simulink model "case7"  (R2024b)
settings: Solver=FixedStepAuto  StartTime=0  StopTime=1  FixedStep=1e-7  RelTol=1e-3
values from neighbouring files (symbols this model uses):
  SG_D_1_D = 0.01056    [IEEE9_case_parameters.m]    (also in case1_parameters.m; case2_parameters.m; case3_parameters.m; case4_parameters.m)
  SG_D_1_EnableSaturation = 0    [IEEE9_case_parameters.m]    (also in case1_parameters.m; case2_parameters.m; case3_parameters.m; case4_parameters.m)
  SG_D_1_f0 = 60    [IEEE9_case_parameters.m]    (also in case1_parameters.m; case2_parameters.m; case3_parameters.m; case4_parameters.m)
  SG_D_1_H = 7.5    [IEEE9_case_parameters.m]    (also in case1_parameters.m; case2_parameters.m; case3_parameters.m; case4_parameters.m)
  SG_D_1_K_A = 20    [IEEE9_case_parameters.m]    (also in case1_parameters.m; case2_parameters.m; case3_parameters.m; case4_parameters.m)
  SG_D_1_K_E = 1.000000e+1    (= 10)    [IEEE9_case_parameters.m]    (also in case1_parameters.m; case2_parameters.m; case3_parameters.m; case4_parameters.m)
  SG_D_1_K_F = 2.363    [IEEE9_case_parameters.m]    (also in case1_parameters.m; case2_parameters.m; case3_parameters.m; case4_parameters.m)
  SG_D_1_K_s = 0.5    [IEEE9_case_parameters.m]    (also in case1_parameters.m = 5; case2_parameters.m = 5; case3_parameters.m = 5; case4_parameters.m = 5)
  SG_D_1_R_a = 0.001088    [IEEE9_case_parameters.m]    (also in case1_parameters.m; case2_parameters.m; case3_parameters.m; case4_parameters.m)
  SG_D_1_S_A = 1    [IEEE9_case_parameters.m]    (also in case1_parameters.m; case2_parameters.m; case3_parameters.m; case4_parameters.m)
  SG_D_1_S_B = 0.103    [IEEE9_case_parameters.m]    (also in case1_parameters.m; case2_parameters.m; case3_parameters.m; case4_parameters.m)
  SG_D_1_S_N = 10.659857    [IEEE9_case_parameters.m]    (also in case1_parameters.m; case2_parameters.m; case3_parameters.m; case4_parameters.m)
  SG_D_1_SpeedPara = 200    [IEEE9_case_parameters.m]    (also in case1_parameters.m; case2_parameters.m; case3_parameters.m; case4_parameters.m)
  SG_D_1_T_0 = 0.720173    [IEEE9_case_parameters.m]    (also in case1_parameters.m = 0.755522; case2_parameters.m = 0.808931; case3_parameters.m = 0.869402; case4_parameters.m = 0.729316)
  SG_D_1_T_1 = 0.3    [IEEE9_case_parameters.m]    (also in case1_parameters.m; case2_parameters.m; case3_parameters.m; case4_parameters.m)
  SG_D_1_T_2 = 0.05    [IEEE9_case_parameters.m]    (also in case1_parameters.m; case2_parameters.m; case3_parameters.m; case4_parameters.m)
  SG_D_1_T_3 = 0.02    [IEEE9_case_parameters.m]    (also in case1_parameters.m; case2_parameters.m; case3_parameters.m; case4_parameters.m)
  SG_D_1_T_4 = 0.005    [IEEE9_case_parameters.m]    (also in case1_parameters.m; case2_parameters.m; case3_parameters.m; case4_parameters.m)
  SG_D_1_T_A = 0.02    [IEEE9_case_parameters.m]    (also in case1_parameters.m; case2_parameters.m; case3_parameters.m; case4_parameters.m)
  SG_D_1_T_dd = 8.000000e+0    (= 8)    [IEEE9_case_parameters.m]    (also in case1_parameters.m; case2_parameters.m; case3_parameters.m; case4_parameters.m)
  SG_D_1_T_ddd = 0.04    [IEEE9_case_parameters.m]    (also in case1_parameters.m; case2_parameters.m; case3_parameters.m; case4_parameters.m)
  SG_D_1_T_E = 0.314    [IEEE9_case_parameters.m]    (also in case1_parameters.m; case2_parameters.m; case3_parameters.m; case4_parameters.m)
  SG_D_1_T_F = 0.35    [IEEE9_case_parameters.m]    (also in case1_parameters.m; case2_parameters.m; case3_parameters.m; case4_parameters.m)
  SG_D_1_T_qd = 0.8    [IEEE9_case_parameters.m]    (also in case1_parameters.m; case2_parameters.m; case3_parameters.m; case4_parameters.m)
  SG_D_1_T_qdd = 0.02    [IEEE9_case_parameters.m]    (also in case1_parameters.m; case2_parameters.m; case3_parameters.m; case4_parameters.m)
  SG_D_1_T_speed = 0.1    [IEEE9_case_parameters.m]    (also in case1_parameters.m = 200; case2_parameters.m = 200; case3_parameters.m = 200; case4_parameters.m = 200)
  SG_D_1_T_w = 0.5    [IEEE9_case_parameters.m]    (also in case1_parameters.m; case2_parameters.m; case3_parameters.m; case4_parameters.m)
  SG_D_1_V_ref = 1.990276    [IEEE9_case_parameters.m]    (also in case1_parameters.m = 2.042296; case2_parameters.m = 2.051388; case3_parameters.m = 2.089584; case4_parameters.m = 2.01845)
  SG_D_1_w_ref = 376.991118    [IEEE9_case_parameters.m]    (also in case1_parameters.m; case2_parameters.m; case3_parameters.m; case4_parameters.m)
  SG_D_1_wb = 6.000000e+1    (= 60)    [IEEE9_case_parameters.m]    (also in case1_parameters.m; case2_parameters.m; case3_parameters.m; case4_parameters.m)
  SG_D_1_x_d = 1.9    [IEEE9_case_parameters.m]    (also in case1_parameters.m; case2_parameters.m; case3_parameters.m; case4_parameters.m)
  SG_D_1_x_dd = 0.302    [IEEE9_case_parameters.m]    (also in case1_parameters.m; case2_parameters.m; case3_parameters.m; case4_parameters.m)
  SG_D_1_x_ddd = 0.204    [IEEE9_case_parameters.m]    (also in case1_parameters.m; case2_parameters.m; case3_parameters.m; case4_parameters.m)
  SG_D_1_x_l = 0.05    [IEEE9_case_parameters.m]    (also in case1_parameters.m; case2_parameters.m; case3_parameters.m; case4_parameters.m)
  SG_D_1_x_q = 1.3    [IEEE9_case_parameters.m]    (also in case1_parameters.m; case2_parameters.m; case3_parameters.m; case4_parameters.m)
  SG_D_1_x_qd = 0.5    [IEEE9_case_parameters.m]    (also in case1_parameters.m; case2_parameters.m; case3_parameters.m; case4_parameters.m)
  SG_D_1_x_qdd = 0.3    [IEEE9_case_parameters.m]    (also in case1_parameters.m; case2_parameters.m; case3_parameters.m; case4_parameters.m)
  SG_D_2_D = 0.02    [IEEE9_case_parameters.m]    (also in case1_parameters.m; case2_parameters.m; case3_parameters.m; case4_parameters.m)
  SG_D_2_EnableSaturation = 0    [IEEE9_case_parameters.m]    (also in case1_parameters.m; case2_parameters.m; case3_parameters.m; case4_parameters.m)
  SG_D_2_f0 = 60    [IEEE9_case_parameters.m]    (also in case1_parameters.m; case2_parameters.m; case3_parameters.m; case4_parameters.m)
  SG_D_2_H = 8.000000e+0    (= 8)    [IEEE9_case_parameters.m]    (also in case1_parameters.m; case2_parameters.m; case3_parameters.m; case4_parameters.m)
  SG_D_2_K_A = 20    [IEEE9_case_parameters.m]    (also in case1_parameters.m; case2_parameters.m; case3_parameters.m; case4_parameters.m)
  SG_D_2_K_E = 1.000000e+1    (= 10)    [IEEE9_case_parameters.m]    (also in case1_parameters.m; case2_parameters.m; case3_parameters.m; case4_parameters.m)
  SG_D_2_K_F = 2.363    [IEEE9_case_parameters.m]    (also in case1_parameters.m; case2_parameters.m; case3_parameters.m; case4_parameters.m)
  SG_D_2_K_s = 0.5    [IEEE9_case_parameters.m]    (also in case1_parameters.m = 4; case2_parameters.m = 4; case3_parameters.m = 4; case4_parameters.m = 4)
  SG_D_2_R_a = 0.001088    [IEEE9_case_parameters.m]    (also in case1_parameters.m; case2_parameters.m; case3_parameters.m; case4_parameters.m)
  SG_D_2_S_A = 1    [IEEE9_case_parameters.m]    (also in case1_parameters.m; case2_parameters.m; case3_parameters.m; case4_parameters.m)
  SG_D_2_S_B = 0.103    [IEEE9_case_parameters.m]    (also in case1_parameters.m; case2_parameters.m; case3_parameters.m; case4_parameters.m)
  SG_D_2_S_N = 10.659857    [IEEE9_case_parameters.m]    (also in case1_parameters.m; case2_parameters.m; case3_parameters.m; case4_parameters.m)
  SG_D_2_SpeedPara = 200    [IEEE9_case_parameters.m]    (also in case1_parameters.m; case2_parameters.m; case3_parameters.m; case4_parameters.m)
  SG_D_2_T_0 = 1.632913    [IEEE9_case_parameters.m]    (also in case1_parameters.m = 1.632925; case2_parameters.m = 1.632915; case3_parameters.m = 1.632914; case4_parameters.m = 1.632927)
  SG_D_2_T_1 = 0.2    [IEEE9_case_parameters.m]    (also in case1_parameters.m; case2_parameters.m; case3_parameters.m; case4_parameters.m)
  SG_D_2_T_2 = 0.05    [IEEE9_case_parameters.m]    (also in case1_parameters.m; case2_parameters.m; case3_parameters.m; case4_parameters.m)
  SG_D_2_T_3 = 0.02    [IEEE9_case_parameters.m]    (also in case1_parameters.m; case2_parameters.m; case3_parameters.m; case4_parameters.m)
  SG_D_2_T_4 = 0.005    [IEEE9_case_parameters.m]    (also in case1_parameters.m; case2_parameters.m; case3_parameters.m; case4_parameters.m)
  SG_D_2_T_A = 0.02    [IEEE9_case_parameters.m]    (also in case1_parameters.m; case2_parameters.m; case3_parameters.m; case4_parameters.m)
  SG_D_2_T_dd = 7.9    [IEEE9_case_parameters.m]    (also in case1_parameters.m; case2_parameters.m; case3_parameters.m; case4_parameters.m)
  SG_D_2_T_ddd = 0.04    [IEEE9_case_parameters.m]    (also in case1_parameters.m; case2_parameters.m; case3_parameters.m; case4_parameters.m)
  SG_D_2_T_E = 0.314    [IEEE9_case_parameters.m]    (also in case1_parameters.m; case2_parameters.m; case3_parameters.m; case4_parameters.m)
  SG_D_2_T_F = 0.35    [IEEE9_case_parameters.m]    (also in case1_parameters.m; case2_parameters.m; case3_parameters.m; case4_parameters.m)
  SG_D_2_T_qd = 0.8    [IEEE9_case_parameters.m]    (also in case1_parameters.m; case2_parameters.m; case3_parameters.m; case4_parameters.m)
  SG_D_2_T_qdd = 0.015    [IEEE9_case_parameters.m]    (also in case1_parameters.m; case2_parameters.m; case3_parameters.m; case4_parameters.m)
  SG_D_2_T_speed = 0.1    [IEEE9_case_parameters.m]    (also in case1_parameters.m = 150; case2_parameters.m = 150; case3_parameters.m = 150; case4_parameters.m = 150)
  SG_D_2_T_w = 0.35    [IEEE9_case_parameters.m]    (also in case1_parameters.m; case2_parameters.m; case3_parameters.m; case4_parameters.m)
  SG_D_2_V_ref = 2.58547    [IEEE9_case_parameters.m]    (also in case1_parameters.m = 2.597896; case2_parameters.m = 2.587136; case3_parameters.m = 2.586042; case4_parameters.m = 2.599679)
  SG_D_2_w_ref = 376.991118    [IEEE9_case_parameters.m]    (also in case1_parameters.m; case2_parameters.m; case3_parameters.m; case4_parameters.m)
  SG_D_2_wb = 6.000000e+1    (= 60)    [IEEE9_case_parameters.m]    (also in case1_parameters.m; case2_parameters.m; case3_parameters.m; case4_parameters.m)
  SG_D_2_x_d = 1.8    [IEEE9_case_parameters.m]    (also in case1_parameters.m; case2_parameters.m; case3_parameters.m; case4_parameters.m)
  SG_D_2_x_dd = 0.302    [IEEE9_case_parameters.m]    (also in case1_parameters.m; case2_parameters.m; case3_parameters.m; case4_parameters.m)
  SG_D_2_x_ddd = 0.204    [IEEE9_case_parameters.m]    (also in case1_parameters.m; case2_parameters.m; case3_parameters.m; case4_parameters.m)
  SG_D_2_x_l = 0.05    [IEEE9_case_parameters.m]    (also in case1_parameters.m; case2_parameters.m; case3_parameters.m; case4_parameters.m)
  SG_D_2_x_q = 1.25    [IEEE9_case_parameters.m]    (also in case1_parameters.m; case2_parameters.m; case3_parameters.m; case4_parameters.m)
  SG_D_2_x_qd = 0.5    [IEEE9_case_parameters.m]    (also in case1_parameters.m; case2_parameters.m; case3_parameters.m; case4_parameters.m)
  SG_D_2_x_qdd = 0.3    [IEEE9_case_parameters.m]    (also in case1_parameters.m; case2_parameters.m; case3_parameters.m; case4_parameters.m)
  SG_D_3_D = 0.02    [IEEE9_case_parameters.m]    (also in case1_parameters.m; case2_parameters.m; case3_parameters.m; case4_parameters.m)
  SG_D_3_EnableSaturation = 0    [IEEE9_case_parameters.m]    (also in case1_parameters.m; case2_parameters.m; case3_parameters.m; case4_parameters.m)
  SG_D_3_f0 = 60    [IEEE9_case_parameters.m]    (also in case1_parameters.m; case2_parameters.m; case3_parameters.m; case4_parameters.m)
  SG_D_3_H = 7.7    [IEEE9_case_parameters.m]    (also in case1_parameters.m; case2_parameters.m; case3_parameters.m; case4_parameters.m)
  SG_D_3_K_A = 20    [IEEE9_case_parameters.m]    (also in case1_parameters.m; case2_parameters.m; case3_parameters.m; case4_parameters.m)
  SG_D_3_K_E = 1.000000e+1    (= 10)    [IEEE9_case_parameters.m]    (also in case1_parameters.m; case2_parameters.m; case3_parameters.m; case4_parameters.m)
  SG_D_3_K_F = 2.363    [IEEE9_case_parameters.m]    (also in case1_parameters.m; case2_parameters.m; case3_parameters.m; case4_parameters.m)
  SG_D_3_K_s = 0.2    [IEEE9_case_parameters.m]    (also in case1_parameters.m = 2; case2_parameters.m = 2; case3_parameters.m = 2; case4_parameters.m = 2)
  SG_D_3_R_a = 0.001088    [IEEE9_case_parameters.m]    (also in case1_parameters.m; case2_parameters.m; case3_parameters.m; case4_parameters.m)
  SG_D_3_S_A = 1    [IEEE9_case_parameters.m]    (also in case1_parameters.m; case2_parameters.m; case3_parameters.m; case4_parameters.m)
  SG_D_3_S_B = 0.103    [IEEE9_case_parameters.m]    (also in case1_parameters.m; case2_parameters.m; case3_parameters.m; case4_parameters.m)
  SG_D_3_S_N = 10.659857    [IEEE9_case_parameters.m]    (also in case1_parameters.m; case2_parameters.m; case3_parameters.m; case4_parameters.m)
  SG_D_3_SpeedPara = 200    [IEEE9_case_parameters.m]    (also in case1_parameters.m; case2_parameters.m; case3_parameters.m; case4_parameters.m)
  SG_D_3_T_0 = 0.850788    [IEEE9_case_parameters.m]    (also in case1_parameters.m = 0.850786; case2_parameters.m = 0.850787; case3_parameters.m; case4_parameters.m = 0.850786)
  SG_D_3_T_1 = 0.2    [IEEE9_case_parameters.m]    (also in case1_parameters.m; case2_parameters.m; case3_parameters.m; case4_parameters.m)
  SG_D_3_T_2 = 0.05    [IEEE9_case_parameters.m]    (also in case1_parameters.m; case2_parameters.m; case3_parameters.m; case4_parameters.m)
  SG_D_3_T_3 = 0.02    [IEEE9_case_parameters.m]    (also in case1_parameters.m; case2_parameters.m; case3_parameters.m; case4_parameters.m)
  SG_D_3_T_4 = 0.005    [IEEE9_case_parameters.m]    (also in case1_parameters.m; case2_parameters.m; case3_parameters.m; case4_parameters.m)
  SG_D_3_T_A = 0.02    [IEEE9_case_parameters.m]    (also in case1_parameters.m; case2_parameters.m; case3_parameters.m; case4_parameters.m)
  SG_D_3_T_dd = 8.1    [IEEE9_case_parameters.m]    (also in case1_parameters.m; case2_parameters.m; case3_parameters.m; case4_parameters.m)
  SG_D_3_T_ddd = 0.04    [IEEE9_case_parameters.m]    (also in case1_parameters.m; case2_parameters.m; case3_parameters.m; case4_parameters.m)
  SG_D_3_T_E = 0.314    [IEEE9_case_parameters.m]    (also in case1_parameters.m; case2_parameters.m; case3_parameters.m; case4_parameters.m)
  SG_D_3_T_F = 0.35    [IEEE9_case_parameters.m]    (also in case1_parameters.m; case2_parameters.m; case3_parameters.m; case4_parameters.m)
  SG_D_3_T_qd = 0.8    [IEEE9_case_parameters.m]    (also in case1_parameters.m; case2_parameters.m; case3_parameters.m; case4_parameters.m)
  SG_D_3_T_qdd = 0.015    [IEEE9_case_parameters.m]    (also in case1_parameters.m; case2_parameters.m; case3_parameters.m; case4_parameters.m)
  SG_D_3_T_speed = 0.1    [IEEE9_case_parameters.m]    (also in case1_parameters.m = 180; case2_parameters.m = 180; case3_parameters.m = 180; case4_parameters.m = 180)
  SG_D_3_T_w = 0.4    [IEEE9_case_parameters.m]    (also in case1_parameters.m; case2_parameters.m; case3_parameters.m; case4_parameters.m)
  SG_D_3_V_ref = 1.892727    [IEEE9_case_parameters.m]    (also in case1_parameters.m = 1.906439; case2_parameters.m = 1.895535; case3_parameters.m = 1.892105; case4_parameters.m = 1.906598)
  SG_D_3_w_ref = 376.991118    [IEEE9_case_parameters.m]    (also in case1_parameters.m; case2_parameters.m; case3_parameters.m; case4_parameters.m)
  SG_D_3_wb = 6.000000e+1    (= 60)    [IEEE9_case_parameters.m]    (also in case1_parameters.m; case2_parameters.m; case3_parameters.m; case4_parameters.m)
  SG_D_3_x_d = 1.85    [IEEE9_case_parameters.m]    (also in case1_parameters.m; case2_parameters.m; case3_parameters.m; case4_parameters.m)
  SG_D_3_x_dd = 0.302    [IEEE9_case_parameters.m]    (also in case1_parameters.m; case2_parameters.m; case3_parameters.m; case4_parameters.m)
  SG_D_3_x_ddd = 0.204    [IEEE9_case_parameters.m]    (also in case1_parameters.m; case2_parameters.m; case3_parameters.m; case4_parameters.m)
  SG_D_3_x_l = 0.05    [IEEE9_case_parameters.m]    (also in case1_parameters.m; case2_parameters.m; case3_parameters.m; case4_parameters.m)
  SG_D_3_x_q = 1.2    [IEEE9_case_parameters.m]    (also in case1_parameters.m; case2_parameters.m; case3_parameters.m; case4_parameters.m)
  SG_D_3_x_qd = 0.5    [IEEE9_case_parameters.m]    (also in case1_parameters.m; case2_parameters.m; case3_parameters.m; case4_parameters.m)
  SG_D_3_x_qdd = 0.3    [IEEE9_case_parameters.m]    (also in case1_parameters.m; case2_parameters.m; case3_parameters.m; case4_parameters.m)
(part 4 of 12)

== system case7/AC_1/d_vq_bus_7_block ==
  note: d_vq_bus_7 in case7
      | $2106.09563369148\,\mathrm{iq}_{\mathrm{bus},7}-376.991118430775\,\mathrm{vd}_{\mathrm{bus},7}$
      | Automatically generated on 2025-10-31 19:27:14 .
  Alge_iq_bus_7_6c77e : Inport
  State_vd_bus_7_c0edf : Inport  Port=2
  Constant_2106.09563369148_c22c3 : Constant  Value=2106.09563369148
  Constant_376.991118430775_b78ad : Constant  Value=376.991118430775
  Product_08e92 : Product
  Product_2e90c : Product
  Subtract_efe12 : Sum  Inputs=+-
  Blockout_d_vq_bus_7_c9af2 : Outport
  wires:
  Constant_2106.09563369148_c22c3/1 -> Product_2e90c/1
  Product_08e92/1 -> Subtract_efe12/2
  Alge_iq_bus_7_6c77e/1 -> Product_2e90c/2
  Constant_376.991118430775_b78ad/1 -> Product_08e92/1
  Subtract_efe12/1 -> Blockout_d_vq_bus_7_c9af2/1
  State_vd_bus_7_c0edf/1 -> Product_08e92/2
  Product_2e90c/1 -> Subtract_efe12/1

== system case7/AC_1/d_vq_bus_8_block ==
  note: d_vq_bus_8 in case7
      | $1657.10381727813\,\mathrm{iq}_{\mathrm{bus},8}-376.991118430775\,\mathrm{vd}_{\mathrm{bus},8}$
      | Automatically generated on 2025-10-31 19:27:16 .
  Alge_iq_bus_8_b3710 : Inport
  State_vd_bus_8_12b43 : Inport  Port=2
  Constant_1657.10381727813_46e6f : Constant  Value=1657.10381727813
  Constant_376.991118430775_a10c9 : Constant  Value=376.991118430775
  Product_577b0 : Product
  Product_c9932 : Product
  Subtract_67862 : Sum  Inputs=+-
  Blockout_d_vq_bus_8_09663 : Outport
  wires:
  Constant_1657.10381727813_46e6f/1 -> Product_577b0/1
  Constant_376.991118430775_a10c9/1 -> Product_c9932/1
  Alge_iq_bus_8_b3710/1 -> Product_577b0/2
  State_vd_bus_8_12b43/1 -> Product_c9932/2
  Product_577b0/1 -> Subtract_67862/1
  Product_c9932/1 -> Subtract_67862/2
  Subtract_67862/1 -> Blockout_d_vq_bus_8_09663/1

== system case7/AC_1/d_vq_bus_9_block ==
  note: d_vq_bus_9 in case7
      | $1564.27849971276\,\mathrm{iq}_{\mathrm{bus},9}-376.991118430775\,\mathrm{vd}_{\mathrm{bus},9}$
      | Automatically generated on 2025-10-31 19:27:19 .
  Alge_iq_bus_9_a8f96 : Inport
  State_vd_bus_9_2f8b2 : Inport  Port=2
  Constant_1564.27849971276_a9894 : Constant  Value=1564.27849971276
  Constant_376.991118430775_a939a : Constant  Value=376.991118430775
  Product_678dc : Product
  Product_f03d7 : Product
  Subtract_bc8b5 : Sum  Inputs=+-
  Blockout_d_vq_bus_9_31261 : Outport
  wires:
  Constant_1564.27849971276_a9894/1 -> Product_f03d7/1
  Constant_376.991118430775_a939a/1 -> Product_678dc/1
  Alge_iq_bus_9_a8f96/1 -> Product_f03d7/2
  State_vd_bus_9_2f8b2/1 -> Product_678dc/2
  Product_f03d7/1 -> Subtract_bc8b5/1
  Product_678dc/1 -> Subtract_bc8b5/2
  Subtract_bc8b5/1 -> Blockout_d_vq_bus_9_31261/1

== system case7/AC_1/id_bus_1_block ==
  note: id_bus_1 in case7
      | $\mathrm{id}_{\mathrm{SG},D,1}-\mathrm{id}_{\mathrm{line},1,4}$
      | Automatically generated on 2025-10-31 19:28:04 .
  Input_id_SG_D_1_eabc6 : Inport
  State_id_line_1_4_aab97 : Inport  Port=2
  Subtract_4393a : Sum  Inputs=+-
  Blockout_id_bus_1_e0036 : Outport
  wires:
  Input_id_SG_D_1_eabc6/1 -> Subtract_4393a/1
  State_id_line_1_4_aab97/1 -> Subtract_4393a/2
  Subtract_4393a/1 -> Blockout_id_bus_1_e0036/1

== system case7/AC_1/id_bus_2_block ==
  note: id_bus_2 in case7
      | $\mathrm{id}_{\mathrm{SG},D,2}+\mathrm{id}_{\mathrm{line},8,2}$
      | Automatically generated on 2025-10-31 19:28:08 .
  Input_id_SG_D_2_cbeb2 : Inport
  State_id_line_8_2_ddc5d : Inport  Port=2
  Add_5b75e : Sum
  Blockout_id_bus_2_1dfd8 : Outport
  wires:
  Input_id_SG_D_2_cbeb2/1 -> Add_5b75e/1
  State_id_line_8_2_ddc5d/1 -> Add_5b75e/2
  Add_5b75e/1 -> Blockout_id_bus_2_1dfd8/1

== system case7/AC_1/id_bus_3_block ==
  note: id_bus_3 in case7
      | $\mathrm{id}_{\mathrm{SG},D,3}-\mathrm{id}_{\mathrm{line},3,6}$
      | Automatically generated on 2025-10-31 19:28:12 .
  Input_id_SG_D_3_5761d : Inport
  State_id_line_3_6_23ff0 : Inport  Port=2
  Subtract_5b783 : Sum  Inputs=+-
  Blockout_id_bus_3_ffcf5 : Outport
  wires:
  Input_id_SG_D_3_5761d/1 -> Subtract_5b783/1
  State_id_line_3_6_23ff0/1 -> Subtract_5b783/2
  Subtract_5b783/1 -> Blockout_id_bus_3_ffcf5/1

== system case7/AC_1/id_bus_4_block ==
  note: id_bus_4 in case7
      | $\mathrm{id}_{\mathrm{line},1,4}-\mathrm{id}_{\mathrm{line},4,5}+\mathrm{id}_{\mathrm{line},9,4}$
      | Automatically generated on 2025-10-31 19:28:14 .
  State_id_line_1_4_3a3fb : Inport
  State_id_line_4_5_64512 : Inport  Port=2
  State_id_line_9_4_0d956 : Inport  Port=3
  Add_d04b2 : Sum
  Subtract_5520f : Sum  Inputs=+-
  Blockout_id_bus_4_096f4 : Outport
  wires:
  State_id_line_9_4_0d956/1 -> Add_d04b2/2
  State_id_line_1_4_3a3fb/1 -> Subtract_5520f/1
  State_id_line_4_5_64512/1 -> Subtract_5520f/2
  Subtract_5520f/1 -> Add_d04b2/1
  Add_d04b2/1 -> Blockout_id_bus_4_096f4/1

== system case7/AC_1/id_bus_5_block ==
  note: id_bus_5 in case7
      | $\mathrm{id}_{\mathrm{line},4,5}-\mathrm{id}_{\mathrm{load},5}-\mathrm{id}_{\mathrm{line},5,6}$
      | Automatically generated on 2025-10-31 19:28:16 .
  State_id_load_5_a1fc8 : Inport
  State_id_line_4_5_aeb7d : Inport  Port=2
  State_id_line_5_6_7e5e7 : Inport  Port=3
  Add_d6f2a : Sum
  Constant_-1_2d1af : Constant  Value=-1
  Product_7594e : Product
  Subtract_9d0cf : Sum  Inputs=+-
  Blockout_id_bus_5_d8728 : Outport
  wires:
  Subtract_9d0cf/1 -> Blockout_id_bus_5_d8728/1
  State_id_line_4_5_aeb7d/1 -> Add_d6f2a/2
  Constant_-1_2d1af/1 -> Product_7594e/1
  Add_d6f2a/1 -> Subtract_9d0cf/1
  State_id_load_5_a1fc8/1 -> Product_7594e/2
  Product_7594e/1 -> Add_d6f2a/1
  State_id_line_5_6_7e5e7/1 -> Subtract_9d0cf/2

== system case7/AC_1/id_bus_6_block ==
  note: id_bus_6 in case7
      | $\mathrm{id}_{\mathrm{line},3,6}+\mathrm{id}_{\mathrm{line},5,6}-\mathrm{id}_{\mathrm{line},6,7}$
      | Automatically generated on 2025-10-31 19:28:18 .
  State_id_line_3_6_b6780 : Inport
  State_id_line_5_6_2d0d9 : Inport  Port=2
  State_id_line_6_7_41759 : Inport  Port=3
  Add_e2ec4 : Sum
  Subtract_1dfb6 : Sum  Inputs=+-
  Blockout_id_bus_6_34f1f : Outport
  wires:
  State_id_line_6_7_41759/1 -> Subtract_1dfb6/2
  State_id_line_3_6_b6780/1 -> Add_e2ec4/1
  State_id_line_5_6_2d0d9/1 -> Add_e2ec4/2
  Add_e2ec4/1 -> Subtract_1dfb6/1
  Subtract_1dfb6/1 -> Blockout_id_bus_6_34f1f/1

== system case7/AC_1/id_bus_7_block ==
  note: id_bus_7 in case7
      | $\mathrm{id}_{\mathrm{line},6,7}-\mathrm{id}_{\mathrm{load},7}-\mathrm{id}_{\mathrm{line},7,8}$
      | Automatically generated on 2025-10-31 19:28:20 .
  State_id_load_7_264fa : Inport
  State_id_line_6_7_22f92 : Inport  Port=2
  State_id_line_7_8_244b4 : Inport  Port=3
  Add_ca084 : Sum
  Constant_-1_8693b : Constant  Value=-1
  Product_5b7d9 : Product
  Subtract_8746d : Sum  Inputs=+-
  Blockout_id_bus_7_f40f2 : Outport
  wires:
  Subtract_8746d/1 -> Blockout_id_bus_7_f40f2/1
  State_id_line_6_7_22f92/1 -> Add_ca084/2
  Constant_-1_8693b/1 -> Product_5b7d9/1
  Add_ca084/1 -> Subtract_8746d/1
  State_id_load_7_264fa/1 -> Product_5b7d9/2
  Product_5b7d9/1 -> Add_ca084/1
  State_id_line_7_8_244b4/1 -> Subtract_8746d/2

== system case7/AC_1/id_bus_8_block ==
  note: id_bus_8 in case7
      | $\mathrm{id}_{\mathrm{line},7,8}-\mathrm{id}_{\mathrm{line},8,2}-\mathrm{id}_{\mathrm{line},8,9}$
      | Automatically generated on 2025-10-31 19:28:23 .
  State_id_line_7_8_e0e98 : Inport
  State_id_line_8_2_e2197 : Inport  Port=2
  State_id_line_8_9_6c8e7 : Inport  Port=3
  Subtract_1c8c3 : Sum  Inputs=+-
  Subtract_aa105 : Sum  Inputs=+-
  Blockout_id_bus_8_dcf1d : Outport
  wires:
  State_id_line_8_9_6c8e7/1 -> Subtract_aa105/2
  State_id_line_7_8_e0e98/1 -> Subtract_1c8c3/1
  State_id_line_8_2_e2197/1 -> Subtract_1c8c3/2
  Subtract_1c8c3/1 -> Subtract_aa105/1
  Subtract_aa105/1 -> Blockout_id_bus_8_dcf1d/1

== system case7/AC_1/id_bus_9_block ==
  note: id_bus_9 in case7
      | $\mathrm{id}_{\mathrm{line},8,9}-\mathrm{id}_{\mathrm{load},9}-\mathrm{id}_{\mathrm{line},9,4}$
      | Automatically generated on 2025-10-31 19:28:25 .
  State_id_load_9_bf11f : Inport
  State_id_line_8_9_50722 : Inport  Port=2
  State_id_line_9_4_40117 : Inport  Port=3
  Add_348e1 : Sum
  Constant_-1_413c0 : Constant  Value=-1
  Product_27b0f : Product
  Subtract_5cca6 : Sum  Inputs=+-
  Blockout_id_bus_9_4ad6a : Outport
  wires:
  Subtract_5cca6/1 -> Blockout_id_bus_9_4ad6a/1
  State_id_line_8_9_50722/1 -> Add_348e1/2
  Constant_-1_413c0/1 -> Product_27b0f/1
  Add_348e1/1 -> Subtract_5cca6/1
  State_id_load_9_bf11f/1 -> Product_27b0f/2
  Product_27b0f/1 -> Add_348e1/1
  State_id_line_9_4_40117/1 -> Subtract_5cca6/2

== system case7/AC_1/iq_bus_1_block ==
  note: iq_bus_1 in case7
      | $\mathrm{iq}_{\mathrm{SG},D,1}-\mathrm{iq}_{\mathrm{line},1,4}$
      | Automatically generated on 2025-10-31 19:28:05 .
  Input_iq_SG_D_1_419da : Inport
  State_iq_line_1_4_cde6a : Inport  Port=2
  Subtract_68868 : Sum  Inputs=+-
  Blockout_iq_bus_1_23a9f : Outport
  wires:
  Input_iq_SG_D_1_419da/1 -> Subtract_68868/1
  State_iq_line_1_4_cde6a/1 -> Subtract_68868/2
  Subtract_68868/1 -> Blockout_iq_bus_1_23a9f/1

== system case7/AC_1/iq_bus_2_block ==
  note: iq_bus_2 in case7
      | $\mathrm{iq}_{\mathrm{SG},D,2}+\mathrm{iq}_{\mathrm{line},8,2}$
      | Automatically generated on 2025-10-31 19:28:09 .
  Input_iq_SG_D_2_9dccc : Inport
  State_iq_line_8_2_f6d21 : Inport  Port=2
  Add_07ce0 : Sum
  Blockout_iq_bus_2_f07a2 : Outport
  wires:
  Input_iq_SG_D_2_9dccc/1 -> Add_07ce0/1
  State_iq_line_8_2_f6d21/1 -> Add_07ce0/2
  Add_07ce0/1 -> Blockout_iq_bus_2_f07a2/1

== system case7/AC_1/iq_bus_3_block ==
  note: iq_bus_3 in case7
      | $\mathrm{iq}_{\mathrm{SG},D,3}-\mathrm{iq}_{\mathrm{line},3,6}$
      | Automatically generated on 2025-10-31 19:28:13 .
  Input_iq_SG_D_3_c42e5 : Inport
  State_iq_line_3_6_82adc : Inport  Port=2
  Subtract_76832 : Sum  Inputs=+-
  Blockout_iq_bus_3_7920f : Outport
  wires:
  Input_iq_SG_D_3_c42e5/1 -> Subtract_76832/1
  State_iq_line_3_6_82adc/1 -> Subtract_76832/2
  Subtract_76832/1 -> Blockout_iq_bus_3_7920f/1

== system case7/AC_1/iq_bus_4_block ==
  note: iq_bus_4 in case7
      | $\mathrm{iq}_{\mathrm{line},1,4}-\mathrm{iq}_{\mathrm{line},4,5}+\mathrm{iq}_{\mathrm{line},9,4}$
      | Automatically generated on 2025-10-31 19:28:15 .
  State_iq_line_1_4_6e840 : Inport
  State_iq_line_4_5_67a6b : Inport  Port=2
  State_iq_line_9_4_bc136 : Inport  Port=3
  Add_d19bc : Sum
  Subtract_43078 : Sum  Inputs=+-
  Blockout_iq_bus_4_5b7f0 : Outport
  wires:
  State_iq_line_1_4_6e840/1 -> Subtract_43078/1
  State_iq_line_4_5_67a6b/1 -> Subtract_43078/2
  Subtract_43078/1 -> Add_d19bc/1
  State_iq_line_9_4_bc136/1 -> Add_d19bc/2
  Add_d19bc/1 -> Blockout_iq_bus_4_5b7f0/1

== system case7/AC_1/iq_bus_5_block ==
  note: iq_bus_5 in case7
      | $\mathrm{iq}_{\mathrm{line},4,5}-\mathrm{iq}_{\mathrm{load},5}-\mathrm{iq}_{\mathrm{line},5,6}$
      | Automatically generated on 2025-10-31 19:28:17 .
  State_iq_load_5_f86bc : Inport
  State_iq_line_4_5_93363 : Inport  Port=2
  State_iq_line_5_6_43169 : Inport  Port=3
  Add_32bb9 : Sum
  Constant_-1_d5412 : Constant  Value=-1
  Product_94716 : Product
  Subtract_7acf6 : Sum  Inputs=+-
  Blockout_iq_bus_5_1d005 : Outport
  wires:
  Subtract_7acf6/1 -> Blockout_iq_bus_5_1d005/1
  State_iq_line_4_5_93363/1 -> Add_32bb9/2
  Constant_-1_d5412/1 -> Product_94716/1
  State_iq_load_5_f86bc/1 -> Product_94716/2
  Product_94716/1 -> Add_32bb9/1
  Add_32bb9/1 -> Subtract_7acf6/1
  State_iq_line_5_6_43169/1 -> Subtract_7acf6/2

== system case7/AC_1/iq_bus_6_block ==
  note: iq_bus_6 in case7
      | $\mathrm{iq}_{\mathrm{line},3,6}+\mathrm{iq}_{\mathrm{line},5,6}-\mathrm{iq}_{\mathrm{line},6,7}$
      | Automatically generated on 2025-10-31 19:28:19 .
  State_iq_line_3_6_53eaa : Inport
  State_iq_line_5_6_87c1e : Inport  Port=2
  State_iq_line_6_7_e327a : Inport  Port=3
  Add_19bb9 : Sum
  Subtract_e9880 : Sum  Inputs=+-
  Blockout_iq_bus_6_0cb61 : Outport
  wires:
  State_iq_line_3_6_53eaa/1 -> Add_19bb9/1
  State_iq_line_5_6_87c1e/1 -> Add_19bb9/2
  Add_19bb9/1 -> Subtract_e9880/1
  State_iq_line_6_7_e327a/1 -> Subtract_e9880/2
  Subtract_e9880/1 -> Blockout_iq_bus_6_0cb61/1

== system case7/AC_1/iq_bus_7_block ==
  note: iq_bus_7 in case7
      | $\mathrm{iq}_{\mathrm{line},6,7}-\mathrm{iq}_{\mathrm{load},7}-\mathrm{iq}_{\mathrm{line},7,8}$
      | Automatically generated on 2025-10-31 19:28:22 .
  State_iq_load_7_cacac : Inport
  State_iq_line_6_7_1e244 : Inport  Port=2
  State_iq_line_7_8_8c678 : Inport  Port=3
  Add_08d5a : Sum
  Constant_-1_82b11 : Constant  Value=-1
  Product_c20ef : Product
  Subtract_827af : Sum  Inputs=+-
  Blockout_iq_bus_7_f78e5 : Outport
  wires:
  Subtract_827af/1 -> Blockout_iq_bus_7_f78e5/1
  State_iq_line_6_7_1e244/1 -> Add_08d5a/2
  Constant_-1_82b11/1 -> Product_c20ef/1
  State_iq_load_7_cacac/1 -> Product_c20ef/2
  Product_c20ef/1 -> Add_08d5a/1
  Add_08d5a/1 -> Subtract_827af/1
  State_iq_line_7_8_8c678/1 -> Subtract_827af/2

== system case7/AC_1/iq_bus_8_block ==
  note: iq_bus_8 in case7
      | $\mathrm{iq}_{\mathrm{line},7,8}-\mathrm{iq}_{\mathrm{line},8,2}-\mathrm{iq}_{\mathrm{line},8,9}$
      | Automatically generated on 2025-10-31 19:28:24 .
  State_iq_line_7_8_8361f : Inport
  State_iq_line_8_2_4ece4 : Inport  Port=2
  State_iq_line_8_9_62274 : Inport  Port=3
  Subtract_aaa9d : Sum  Inputs=+-
  Subtract_ba02c : Sum  Inputs=+-
  Blockout_iq_bus_8_3d53c : Outport
  wires:
  State_iq_line_7_8_8361f/1 -> Subtract_aaa9d/1
  State_iq_line_8_2_4ece4/1 -> Subtract_aaa9d/2
  Subtract_aaa9d/1 -> Subtract_ba02c/1
  State_iq_line_8_9_62274/1 -> Subtract_ba02c/2
  Subtract_ba02c/1 -> Blockout_iq_bus_8_3d53c/1

== system case7/AC_1/iq_bus_9_block ==
  note: iq_bus_9 in case7
      | $\mathrm{iq}_{\mathrm{line},8,9}-\mathrm{iq}_{\mathrm{load},9}-\mathrm{iq}_{\mathrm{line},9,4}$
      | Automatically generated on 2025-10-31 19:28:26 .
  State_iq_load_9_c0b16 : Inport
  State_iq_line_8_9_e9f4e : Inport  Port=2
  State_iq_line_9_4_2d700 : Inport  Port=3
  Add_3bcab : Sum
  Constant_-1_dbcb5 : Constant  Value=-1
  Product_3b195 : Product
  Subtract_4c0d0 : Sum  Inputs=+-
  Blockout_iq_bus_9_80b8d : Outport
  wires:
  Subtract_4c0d0/1 -> Blockout_iq_bus_9_80b8d/1
  State_iq_line_8_9_e9f4e/1 -> Add_3bcab/2
  Constant_-1_dbcb5/1 -> Product_3b195/1
  State_iq_load_9_c0b16/1 -> Product_3b195/2
  Product_3b195/1 -> Add_3bcab/1
  Add_3bcab/1 -> Subtract_4c0d0/1
  State_iq_line_9_4_2d700/1 -> Subtract_4c0d0/2

== system case7/AC_1/vd_bus_1_out_block ==
  note: vd_bus_1_out in case7
      | $\mathrm{vd}_{\mathrm{bus},1}$
      | Automatically generated on 2025-10-31 19:28:02 .
  State_vd_bus_1_3d051 : Inport
  Blockout_vd_bus_1_out_c0c69 : Outport
  wires:
  State_vd_bus_1_3d051/1 -> Blockout_vd_bus_1_out_c0c69/1

== system case7/AC_1/vd_bus_2_out_block ==
  note: vd_bus_2_out in case7
      | $\mathrm{vd}_{\mathrm{bus},2}$
      | Automatically generated on 2025-10-31 19:28:06 .
  State_vd_bus_2_3d298 : Inport
  Blockout_vd_bus_2_out_3aeaa : Outport
  wires:
  State_vd_bus_2_3d298/1 -> Blockout_vd_bus_2_out_3aeaa/1

== system case7/AC_1/vd_bus_3_out_block ==
  note: vd_bus_3_out in case7
      | $\mathrm{vd}_{\mathrm{bus},3}$
      | Automatically generated on 2025-10-31 19:28:10 .
  State_vd_bus_3_0fcd0 : Inport
  Blockout_vd_bus_3_out_587ae : Outport
  wires:
  State_vd_bus_3_0fcd0/1 -> Blockout_vd_bus_3_out_587ae/1

== system case7/AC_1/vq_bus_1_out_block ==
  note: vq_bus_1_out in case7
      | $\mathrm{vq}_{\mathrm{bus},1}$
      | Automatically generated on 2025-10-31 19:28:03 .
  State_vq_bus_1_e6f2a : Inport
  Blockout_vq_bus_1_out_89e60 : Outport
  wires:
  State_vq_bus_1_e6f2a/1 -> Blockout_vq_bus_1_out_89e60/1

== system case7/AC_1/vq_bus_2_out_block ==
  note: vq_bus_2_out in case7
      | $\mathrm{vq}_{\mathrm{bus},2}$
      | Automatically generated on 2025-10-31 19:28:07 .
  State_vq_bus_2_798f2 : Inport
  Blockout_vq_bus_2_out_5c378 : Outport
  wires:
  State_vq_bus_2_798f2/1 -> Blockout_vq_bus_2_out_5c378/1

== system case7/AC_1/vq_bus_3_out_block ==
  note: vq_bus_3_out in case7
      | $\mathrm{vq}_{\mathrm{bus},3}$
      | Automatically generated on 2025-10-31 19:28:11 .
  State_vq_bus_3_a3a16 : Inport
  Blockout_vq_bus_3_out_91852 : Outport
  wires:
  State_vq_bus_3_a3a16/1 -> Blockout_vq_bus_3_out_91852/1

== system case7/SG_D_1/T_e_SG_D_1_block ==
  note: T_e_SG_D_1 in case7
      | $-\frac{\psi _{d,\mathrm{SG},D,1}\,\left(\psi _{q,\mathrm{SG},D,1}+\frac{\psi _{\mathrm{gq},\mathrm{SG},D,1}\,\left(x_{l}-x_{\mathrm{qdd}}\right)}{x_{l}-x_{\mathrm{qd}}}+\frac{\psi _{\mathrm{kq},\mathrm{SG},D,1}\,\left(x_{\mathrm{qd}}-x_{\mathrm{qdd}}\right)}{x_{l}-x_{\mathrm{qd}}}\right)}{x_{\mathrm{qdd}}}-\frac{\psi _{q,\mathrm{SG},D,1}\,\left(\frac{\psi _{\mathrm{1d},\mathrm{SG},D,1}\,\left(x_{\mathrm{dd}}-x_{\mathrm{ddd}}\right)}{x_{\mathrm{dd}}-x_{l}}-\psi _{d,\mathrm{SG},D,1}+\frac{\psi _{\mathrm{fd},\mathrm{SG},D,1}\,\left(x_{\mathrm{ddd}}-x_{l}\right)}{x_{\mathrm{dd}}-x_{l}}\right)}{x_{\mathrm{ddd}}}$
      | Automatically generated on 2025-10-31 19:23:57 .
  State_psi_d_SG_D_1_a3ce0 : Inport
  State_psi_gq_SG_D_1_d5669 : Inport  Port=2
  State_psi_kq_SG_D_1_0bf11 : Inport  Port=3
  State_psi_q_SG_D_1_4e8fb : Inport  Port=4
  State_psi_q_SG_D_1_74d13 : Inport  Port=5
  State_psi_1d_SG_D_1_b5c2d : Inport  Port=6
  State_psi_d_SG_D_1_70569 : Inport  Port=7
  State_psi_fd_SG_D_1_5c3bd : Inport  Port=8
  Add_68c9d : Sum
  Add_79f0a : Sum
  Add_7aecc : Sum
  Add_8ee55 : Sum
  Add_ce113 : Sum
  Add_e0855 : Sum
  Constant_-1_14969 : Constant  Value=-1
  Constant_-1_31aec : Constant  Value=-1
  Constant_-1_85a2e : Constant  Value=-1
  Constant_-1_9c5b0 : Constant  Value=-1
  Constant_-1_a1e35 : Constant  Value=-1
  Constant_x_dd_0b8d7 : Constant  Value=x_dd
  Constant_x_dd_6a894 : Constant  Value=x_dd
  Constant_x_dd_c329e : Constant  Value=x_dd
  Constant_x_ddd_20e4e : Constant  Value=x_ddd
  Constant_x_ddd_85732 : Constant  Value=x_ddd
  Constant_x_ddd_c2fd5 : Constant  Value=x_ddd
  Constant_x_l_20241 : Constant  Value=x_l
  Constant_x_l_213a2 : Constant  Value=x_l
  Constant_x_l_6007d : Constant  Value=x_l
  Constant_x_l_63fef : Constant  Value=x_l
  Constant_x_l_b515a : Constant  Value=x_l
  Constant_x_l_fe346 : Constant  Value=x_l
  Constant_x_qd_521ff : Constant  Value=x_qd
  Constant_x_qd_76663 : Constant  Value=x_qd
  Constant_x_qd_d56cd : Constant  Value=x_qd
  Constant_x_qdd_bdbc3 : Constant  Value=x_qdd
  Constant_x_qdd_d270e : Constant  Value=x_qdd
  Constant_x_qdd_f1224 : Constant  Value=x_qdd
  Divide_08526 : Product  Inputs=*/
  Divide_608d9 : Product  Inputs=*/
  Divide_7ee6a : Product  Inputs=*/
  Divide_c25e3 : Product  Inputs=*/
  Divide_e5438 : Product  Inputs=*/
  Divide_f104a : Product  Inputs=*/
  Product_49955 : Product
  Product_64f0b : Product
  Product_8dc78 : Product
  Product_96091 : Product
  Product_9f897 : Product
  Product_adb74 : Product
  Product_b9941 : Product
  Product_c681b : Product
  Product_dfaea : Product
  Product_f6843 : Product
  Product_fa03b : Product
  Subtract_05876 : Sum  Inputs=+-
  Subtract_0c5e2 : Sum  Inputs=+-
  Subtract_42aa9 : Sum  Inputs=+-
  Subtract_45933 : Sum  Inputs=+-
  Subtract_47e19 : Sum  Inputs=+-
  Subtract_60a43 : Sum  Inputs=+-
  Subtract_9c084 : Sum  Inputs=+-
  Blockout_T_e_SG_D_1_7d4c7 : Outport
  wires:
  Product_dfaea/1 -> Divide_608d9/1
  Product_fa03b/1 -> Add_e0855/1
  Divide_608d9/1 -> Subtract_05876/1
  Constant_-1_85a2e/1 -> Product_fa03b/1
  Constant_x_l_6007d/1 -> Product_fa03b/2
  Constant_x_qdd_d270e/1 -> Add_e0855/2
  Constant_x_qd_76663/1 -> Subtract_9c084/1
  Constant_-1_14969/1 -> Product_96091/1
  Constant_x_qdd_f1224/1 -> Divide_7ee6a/2
  Constant_x_qdd_bdbc3/1 -> Subtract_9c084/2
  State_psi_q_SG_D_1_74d13/1 -> Product_8dc78/1
  Constant_x_dd_6a894/1 -> Subtract_47e19/1
  Constant_x_l_20241/1 -> Product_96091/2
  Subtract_47e19/1 -> Product_c681b/2
  Constant_-1_a1e35/1 -> Product_64f0b/1
  Constant_x_l_fe346/1 -> Product_64f0b/2
  Subtract_0c5e2/1 -> Product_8dc78/2
  State_psi_q_SG_D_1_4e8fb/1 -> Add_68c9d/2
  Constant_-1_31aec/1 -> Product_adb74/1
  State_psi_1d_SG_D_1_b5c2d/1 -> Product_adb74/2
  Constant_x_ddd_85732/1 -> Subtract_47e19/2
  State_psi_gq_SG_D_1_d5669/1 -> Product_dfaea/1
  Add_e0855/1 -> Product_dfaea/2
  Product_96091/1 -> Add_ce113/1
  Product_b9941/1 -> Product_f6843/1
  Constant_x_qd_d56cd/1 -> Add_ce113/2
  Product_c681b/1 -> Divide_f104a/1
  State_psi_kq_SG_D_1_0bf11/1 -> Product_49955/1
  Add_ce113/1 -> Divide_608d9/2
  Subtract_9c084/1 -> Product_49955/2
  Product_64f0b/1 -> Add_7aecc/1
  Constant_x_qd_521ff/1 -> Add_7aecc/2
  Product_49955/1 -> Divide_e5438/1
  Product_adb74/1 -> Product_c681b/1
  Constant_x_dd_c329e/1 -> Subtract_60a43/1
  Constant_x_l_b515a/1 -> Subtract_60a43/2
  Constant_x_ddd_20e4e/1 -> Subtract_45933/1
  Product_8dc78/1 -> Divide_c25e3/1
  Constant_x_l_213a2/1 -> Subtract_45933/2
  Divide_7ee6a/1 -> Add_79f0a/1
  Product_f6843/1 -> Divide_7ee6a/1
  Add_7aecc/1 -> Divide_e5438/2
  Subtract_05876/1 -> Add_68c9d/1
  Divide_e5438/1 -> Subtract_05876/2
  Subtract_60a43/1 -> Divide_f104a/2
  State_psi_fd_SG_D_1_5c3bd/1 -> Product_9f897/1
  Constant_x_ddd_c2fd5/1 -> Divide_c25e3/2
  Subtract_45933/1 -> Product_9f897/2
  Constant_x_dd_0b8d7/1 -> Subtract_42aa9/1
  Constant_x_l_63fef/1 -> Subtract_42aa9/2
  Divide_f104a/1 -> Add_8ee55/1
  Add_8ee55/1 -> Subtract_0c5e2/1
  State_psi_d_SG_D_1_70569/1 -> Add_8ee55/2
  Product_9f897/1 -> Divide_08526/1
  Subtract_42aa9/1 -> Divide_08526/2
  Constant_-1_9c5b0/1 -> Product_b9941/1
  State_psi_d_SG_D_1_a3ce0/1 -> Product_b9941/2
  Divide_08526/1 -> Subtract_0c5e2/2
  Add_68c9d/1 -> Product_f6843/2
  Divide_c25e3/1 -> Add_79f0a/2
  Add_79f0a/1 -> Blockout_T_e_SG_D_1_7d4c7/1

== system case7/SG_D_1/d_E_fd_SG_D_1_block ==
  note: d_E_fd_SG_D_1 in case7
      | $\frac{V_{f,\mathrm{SG},D,1}-E_{\mathrm{fd},\mathrm{SG},D,1}\,K_{E}}{T_{E}}$
      | Automatically generated on 2025-10-31 19:23:43 .
  State_E_fd_SG_D_1_10d5b : Inport
  State_V_f_SG_D_1_10c68 : Inport  Port=2
  Add_28230 : Sum
  Constant_-1_7fc28 : Constant  Value=-1
  Constant_K_E_7e2f8 : Constant  Value=K_E
  Constant_T_E_3231d : Constant  Value=T_E
  Divide_e1d86 : Product  Inputs=*/
  Product_625f3 : Product
  Product_a21fe : Product
  Blockout_d_E_fd_SG_D_1_39807 : Outport
  wires:
  Add_28230/1 -> Divide_e1d86/1
  Constant_-1_7fc28/1 -> Product_a21fe/1
  State_E_fd_SG_D_1_10d5b/1 -> Product_a21fe/2
  Product_a21fe/1 -> Product_625f3/1
  Constant_K_E_7e2f8/1 -> Product_625f3/2
  Product_625f3/1 -> Add_28230/1
  Constant_T_E_3231d/1 -> Divide_e1d86/2
  State_V_f_SG_D_1_10c68/1 -> Add_28230/2
  Divide_e1d86/1 -> Blockout_d_E_fd_SG_D_1_39807/1

== system case7/SG_D_1/d_Px_1_SG_D_1_block ==
  note: d_Px_1_SG_D_1 in case7
      | $\frac{w_{\mathrm{SG},D,1}-2\,\pi \,f_{0}}{T_{w}}-\frac{\mathrm{Px}_{1,\mathrm{SG},D,1}}{T_{w}}$
      | Automatically generated on 2025-10-31 19:23:44 .
  State_Px_1_SG_D_1_12f8b : Inport
  State_w_SG_D_1_1213f : Inport  Port=2
  Add_58a29 : Sum
  Add_cddc7 : Sum
  Constant_-1_e5479 : Constant  Value=-1
  Constant_-2.0_740f6 : Constant  Value=-2.0
  Constant_T_w_0f2d2 : Constant  Value=T_w
  Constant_T_w_89f6f : Constant  Value=T_w
  Constant_f0_615f2 : Constant  Value=f0
  Constant_pi_d04be : Constant  Value=pi
  Divide_85064 : Product  Inputs=*/
  Divide_f88cc : Product  Inputs=*/
  Product_22bb3 : Product
  Product_de461 : Product
  Product_e3f24 : Product
  Blockout_d_Px_1_SG_D_1_d3439 : Outport
  wires:
  Add_58a29/1 -> Blockout_d_Px_1_SG_D_1_d3439/1
  Constant_-2.0_740f6/1 -> Product_de461/1
  Product_22bb3/1 -> Divide_85064/1
  State_w_SG_D_1_1213f/1 -> Add_cddc7/2
  Constant_-1_e5479/1 -> Product_22bb3/1
  Constant_f0_615f2/1 -> Product_e3f24/2
  Constant_pi_d04be/1 -> Product_de461/2
  Product_e3f24/1 -> Add_cddc7/1
  Product_de461/1 -> Product_e3f24/1
  State_Px_1_SG_D_1_12f8b/1 -> Product_22bb3/2
  Constant_T_w_0f2d2/1 -> Divide_85064/2
  Add_cddc7/1 -> Divide_f88cc/1
  Constant_T_w_89f6f/1 -> Divide_f88cc/2
  Divide_85064/1 -> Add_58a29/1
  Divide_f88cc/1 -> Add_58a29/2

== system case7/SG_D_1/d_Px_2_SG_D_1_block ==
  note: d_Px_2_SG_D_1 in case7
      | $\frac{\mathrm{Px}_{1,\mathrm{SG},D,1}-T_{2}\,\left(\frac{\mathrm{Px}_{1,\mathrm{SG},D,1}}{T_{w}}-\frac{w_{\mathrm{SG},D,1}-2\,\pi \,f_{0}}{T_{w}}\right)}{T_{1}}-\frac{\mathrm{Px}_{2,\mathrm{SG},D,1}}{T_{1}}$
      | Automatically generated on 2025-10-31 19:23:46 .
  State_Px_2_SG_D_1_00b8c : Inport
  State_Px_1_SG_D_1_dc188 : Inport  Port=2
  State_Px_1_SG_D_1_61a1c : Inport  Port=3
  State_w_SG_D_1_9cb57 : Inport  Port=4
  Add_6e969 : Sum
  Add_79f1e : Sum
  Add_a60f8 : Sum
  Add_e66a0 : Sum
  Constant_-1_539e0 : Constant  Value=-1
  Constant_-1_fee56 : Constant  Value=-1
  Constant_-2.0_16e62 : Constant  Value=-2.0
  Constant_T_1_2ff83 : Constant  Value=T_1
  Constant_T_1_4c367 : Constant  Value=T_1
  Constant_T_2_f04a0 : Constant  Value=T_2
  Constant_T_w_baeee : Constant  Value=T_w
  Constant_T_w_bbc0d : Constant  Value=T_w
  Constant_f0_1fd96 : Constant  Value=f0
  Constant_pi_5dd1d : Constant  Value=pi
  Divide_75a8e : Product  Inputs=*/
  Divide_a549b : Product  Inputs=*/
  Divide_ad176 : Product  Inputs=*/
  Divide_adfc3 : Product  Inputs=*/
  Product_1d6e1 : Product
  Product_76c4c : Product
  Product_83d86 : Product
  Product_b9dcb : Product
  Product_d4cfe : Product
  Blockout_d_Px_2_SG_D_1_bbd82 : Outport
  wires:
  Constant_-2.0_16e62/1 -> Product_b9dcb/1
  State_w_SG_D_1_9cb57/1 -> Add_6e969/2
  Constant_f0_1fd96/1 -> Product_76c4c/2
  Constant_pi_5dd1d/1 -> Product_b9dcb/2
  Add_a60f8/1 -> Product_83d86/2
  Product_76c4c/1 -> Add_6e969/1
  Divide_ad176/1 -> Add_a60f8/1
  Product_b9dcb/1 -> Product_76c4c/1
  Constant_T_w_bbc0d/1 -> Divide_ad176/2
  Constant_-1_539e0/1 -> Product_1d6e1/1
  State_Px_1_SG_D_1_61a1c/1 -> Product_1d6e1/2
  Divide_a549b/1 -> Add_79f1e/1
  Product_1d6e1/1 -> Divide_ad176/1
  Add_6e969/1 -> Divide_adfc3/1
  Constant_T_w_baeee/1 -> Divide_adfc3/2
  Divide_adfc3/1 -> Add_a60f8/2
  Constant_T_2_f04a0/1 -> Product_83d86/1
  Constant_-1_fee56/1 -> Product_d4cfe/1
  State_Px_2_SG_D_1_00b8c/1 -> Product_d4cfe/2
  State_Px_1_SG_D_1_dc188/1 -> Add_e66a0/1
  Product_83d86/1 -> Add_e66a0/2
  Add_e66a0/1 -> Divide_75a8e/1
  Product_d4cfe/1 -> Divide_a549b/1
  Constant_T_1_2ff83/1 -> Divide_a549b/2
  Constant_T_1_4c367/1 -> Divide_75a8e/2
  Divide_75a8e/1 -> Add_79f1e/2
  Add_79f1e/1 -> Blockout_d_Px_2_SG_D_1_bbd82/1

== system case7/SG_D_1/d_Px_3_SG_D_1_block ==
  note: d_Px_3_SG_D_1 in case7
      | $\frac{\mathrm{Px}_{2,\mathrm{SG},D,1}+T_{4}\,\left(\frac{\mathrm{Px}_{1,\mathrm{SG},D,1}-T_{2}\,\left(\frac{\mathrm{Px}_{1,\mathrm{SG},D,1}}{T_{w}}-\frac{w_{\mathrm{SG},D,1}-2\,\pi \,f_{0}}{T_{w}}\right)}{T_{1}}-\frac{\mathrm{Px}_{2,\mathrm{SG},D,1}}{T_{1}}\right)}{T_{3}}-\frac{\mathrm{Px}_{3,\mathrm{SG},D,1}}{T_{3}}$
      | Automatically generated on 2025-10-31 19:23:48 .
  State_Px_3_SG_D_1_1460f : Inport
  State_Px_2_SG_D_1_f74b9 : Inport  Port=2
  State_Px_2_SG_D_1_0b119 : Inport  Port=3
  State_Px_1_SG_D_1_9c31b : Inport  Port=4
  State_Px_1_SG_D_1_3806b : Inport  Port=5
  State_w_SG_D_1_58194 : Inport  Port=6
  Add_05708 : Sum
  Add_533c2 : Sum
  Add_b23ba : Sum
  Add_be6d5 : Sum
  Add_fadcd : Sum
  Add_fba52 : Sum
  Constant_-1_3f9f0 : Constant  Value=-1
  Constant_-1_51921 : Constant  Value=-1
  Constant_-1_ae59a : Constant  Value=-1
  Constant_-2.0_5606d : Constant  Value=-2.0
  Constant_T_1_41df7 : Constant  Value=T_1
  Constant_T_1_d6f55 : Constant  Value=T_1
  Constant_T_2_0f5cb : Constant  Value=T_2
  Constant_T_3_af73e : Constant  Value=T_3
  Constant_T_3_c3042 : Constant  Value=T_3
  Constant_T_4_72bdc : Constant  Value=T_4
  Constant_T_w_6cf67 : Constant  Value=T_w
  Constant_T_w_9e242 : Constant  Value=T_w
  Constant_f0_cd506 : Constant  Value=f0
  Constant_pi_d1f43 : Constant  Value=pi
  Divide_35fec : Product  Inputs=*/
  Divide_7ee48 : Product  Inputs=*/
  Divide_8cf26 : Product  Inputs=*/
  Divide_96172 : Product  Inputs=*/
  Divide_9e82d : Product  Inputs=*/
  Divide_a05b4 : Product  Inputs=*/
  Product_52e63 : Product
  Product_5dbb3 : Product
  Product_a324d : Product
  Product_ac74e : Product
  Product_bd2e6 : Product
  Product_e4539 : Product
  Product_efd86 : Product
  Blockout_d_Px_3_SG_D_1_d35bd : Outport
  wires:
  Constant_T_w_9e242/1 -> Divide_9e82d/2
  Constant_-1_51921/1 -> Product_efd86/1
  Add_fba52/1 -> Blockout_d_Px_3_SG_D_1_d35bd/1
  Constant_-2.0_5606d/1 -> Product_e4539/1
  State_w_SG_D_1_58194/1 -> Add_fadcd/2
  Constant_f0_cd506/1 -> Product_bd2e6/2
  State_Px_1_SG_D_1_3806b/1 -> Product_efd86/2
  Constant_pi_d1f43/1 -> Product_e4539/2
  Product_bd2e6/1 -> Add_fadcd/1
  Product_e4539/1 -> Product_bd2e6/1
  Product_efd86/1 -> Divide_9e82d/1
  Divide_7ee48/1 -> Add_fba52/1
  Constant_T_3_c3042/1 -> Divide_8cf26/2
  Add_fadcd/1 -> Divide_35fec/1
  Constant_T_w_6cf67/1 -> Divide_35fec/2
  Divide_9e82d/1 -> Add_05708/1
  Divide_35fec/1 -> Add_05708/2
  Constant_-1_3f9f0/1 -> Product_5dbb3/1
  Constant_T_2_0f5cb/1 -> Product_a324d/1
  Add_05708/1 -> Product_a324d/2
  Constant_-1_ae59a/1 -> Product_52e63/1
  Divide_8cf26/1 -> Add_fba52/2
  Constant_T_3_af73e/1 -> Divide_7ee48/2
  State_Px_2_SG_D_1_0b119/1 -> Product_52e63/2
  State_Px_1_SG_D_1_9c31b/1 -> Add_b23ba/1
  Divide_96172/1 -> Add_533c2/1
  Product_a324d/1 -> Add_b23ba/2
  Product_52e63/1 -> Divide_96172/1
  Product_5dbb3/1 -> Divide_7ee48/1
  Constant_T_1_d6f55/1 -> Divide_96172/2
  Add_b23ba/1 -> Divide_a05b4/1
  Constant_T_1_41df7/1 -> Divide_a05b4/2
  Divide_a05b4/1 -> Add_533c2/2
  Constant_T_4_72bdc/1 -> Product_ac74e/1
  Add_533c2/1 -> Product_ac74e/2
  State_Px_3_SG_D_1_1460f/1 -> Product_5dbb3/2
  State_Px_2_SG_D_1_f74b9/1 -> Add_be6d5/1
  Product_ac74e/1 -> Add_be6d5/2
  Add_be6d5/1 -> Divide_8cf26/1

== system case7/SG_D_1/d_R_f_SG_D_1_block ==
  note: d_R_f_SG_D_1 in case7
      | $-\frac{R_{f,\mathrm{SG},D,1}-\frac{E_{\mathrm{fd},\mathrm{SG},D,1}\,K_{F}}{T_{F}}}{T_{F}}$
      | Automatically generated on 2025-10-31 19:23:42 .
  State_E_fd_SG_D_1_6cf46 : Inport
  State_R_f_SG_D_1_306fb : Inport  Port=2
  Constant_K_F_659ad : Constant  Value=K_F
  Constant_T_F_2f725 : Constant  Value=T_F
  Constant_T_F_4a3ef : Constant  Value=T_F
  Divide_5a834 : Product  Inputs=*/
  Divide_771cd : Product  Inputs=*/
  Product_afb2f : Product
  Subtract_9b5e8 : Sum  Inputs=+-
  Blockout_d_R_f_SG_D_1_0120a : Outport
  wires:
  Constant_K_F_659ad/1 -> Product_afb2f/2
  Product_afb2f/1 -> Divide_771cd/1
  State_E_fd_SG_D_1_6cf46/1 -> Product_afb2f/1
  State_R_f_SG_D_1_306fb/1 -> Subtract_9b5e8/2
  Constant_T_F_2f725/1 -> Divide_771cd/2
  Divide_771cd/1 -> Subtract_9b5e8/1
  Divide_5a834/1 -> Blockout_d_R_f_SG_D_1_0120a/1
  Subtract_9b5e8/1 -> Divide_5a834/1
  Constant_T_F_4a3ef/1 -> Divide_5a834/2

== system case7/SG_D_1/d_T_m_SG_D_1_block ==
  note: d_T_m_SG_D_1 in case7
      | $-\frac{T_{m,\mathrm{SG},D,1}-T_{0}+\frac{\mathrm{SpeedPara}\,\left(w_{\mathrm{SG},D,1}-w_{\mathrm{ref}}\right)}{2\,f_{0}\,\pi }}{T_{\mathrm{speed}}}$
      | Automatically generated on 2025-10-31 19:23:32 .
  State_w_SG_D_1_ed6bc : Inport
  State_T_m_SG_D_1_97fbd : Inport  Port=2
  Add_2f7b8 : Sum
  Add_af414 : Sum
  Constant_-1_b33a5 : Constant  Value=-1
  Constant_2.0_3cd70 : Constant  Value=2.0
  Constant_SpeedPara_10858 : Constant  Value=SpeedPara
  Constant_T_0_04495 : Constant  Value=T_0
  Constant_T_speed_45414 : Constant  Value=T_speed
  Constant_f0_c0163 : Constant  Value=f0
  Constant_pi_2bbad : Constant  Value=pi
  Constant_w_ref_9cf28 : Constant  Value=w_ref
  Divide_7e1be : Product  Inputs=*/
  Divide_8040c : Product  Inputs=*/
  Product_268cf : Product
  Product_5e68d : Product
  Product_7bac7 : Product
  Product_e74dd : Product
  Subtract_95fbe : Sum  Inputs=+-
  Blockout_d_T_m_SG_D_1_03812 : Outport
  wires:
  Constant_-1_b33a5/1 -> Product_7bac7/1
  Constant_w_ref_9cf28/1 -> Add_2f7b8/2
  State_w_SG_D_1_ed6bc/1 -> Product_7bac7/2
  Add_af414/1 -> Subtract_95fbe/1
  Add_2f7b8/1 -> Product_268cf/2
  Product_7bac7/1 -> Add_2f7b8/1
  Constant_2.0_3cd70/1 -> Product_5e68d/1
  Constant_pi_2bbad/1 -> Product_5e68d/2
  Constant_SpeedPara_10858/1 -> Product_268cf/1
  Product_5e68d/1 -> Product_e74dd/1
  Constant_f0_c0163/1 -> Product_e74dd/2
  Constant_T_speed_45414/1 -> Divide_7e1be/2
  Product_268cf/1 -> Divide_8040c/1
  Product_e74dd/1 -> Divide_8040c/2
  Divide_8040c/1 -> Add_af414/1
  Constant_T_0_04495/1 -> Add_af414/2
  State_T_m_SG_D_1_97fbd/1 -> Subtract_95fbe/2
  Subtract_95fbe/1 -> Divide_7e1be/1
  Divide_7e1be/1 -> Blockout_d_T_m_SG_D_1_03812/1
